simulink model "controller"  (R2023b)
settings: Solver=VariableStepAuto  StartTime=0.0  StopTime=10.0  RelTol=1e-3
undefined symbols (not defined in the file or in its folder): u0, u_lim_max, u_lim_min
settings Model: Creator=fabioschneider  LastModifiedBy=fabioschneider
settings DebuggingCC: ModelReferenceExtraNoncontSigs=none

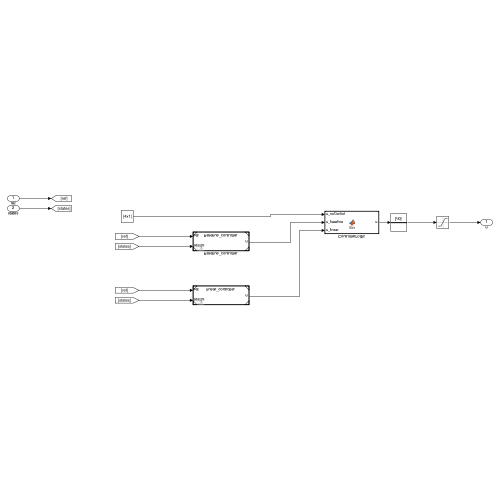
[thumbnail: Simulink's stored preview of the top-level diagram]
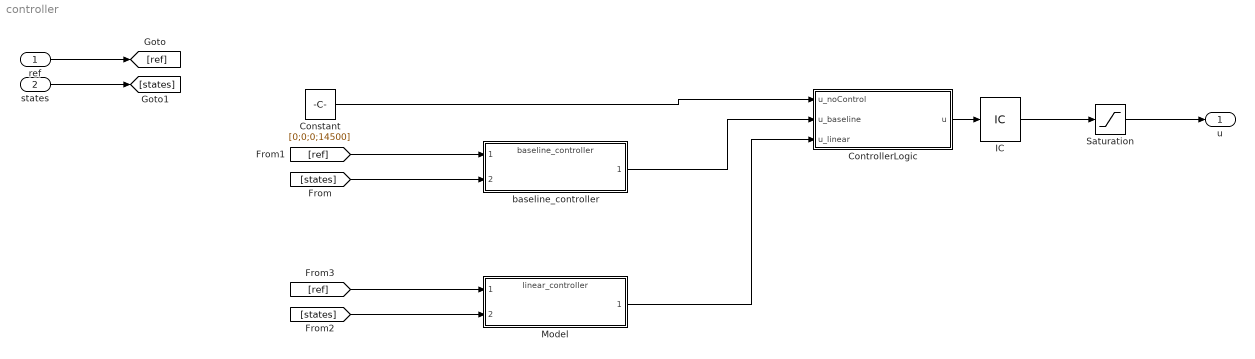
== system controller ==
  ref : Inport
  states : Inport  Port=2
  Constant : Constant  Value=[0;0;0;14500]  SampleTime=-1
  ControllerLogic : MATLAB Function  TreatAsAtomicUnit=on
  IC : InitialCondition  Value=u0
  Model : ModelReference  ModelNameDialog=linear_controller.slx  SimulationMode=Normal  ModelReferenceVersion=1.9
  Saturation : Saturate  UpperLimit=u_lim_max  LowerLimit=u_lim_min
  baseline_controller : ModelReference  ModelNameDialog=baseline_controller.slx  SimulationMode=Normal  ModelReferenceVersion=1.13
  u : Outport
  wires:
  ControllerLogic/1(u) -> IC/1
  Constant/1 -> ControllerLogic/1(u_noControl)
  baseline_controller/1 -> ControllerLogic/2(u_baseline)
  ref/1 -> [ref]
  states/1 -> [states]
  [states] -> baseline_controller/2
  [ref] -> baseline_controller/1
  Model/1 -> ControllerLogic/3(u_linear)
  IC/1 -> Saturation/1
  [ref] -> Model/1
  [states] -> Model/2
  Saturation/1 -> u/1

== matlab function controller/ControllerLogic ==
  data: u_noControl input; u output; u_baseline input; u_linear input; activeController parameter
function u = fcn(u_noControl, u_baseline, u_linear, activeController)

u = controller_logic(u_noControl, u_baseline, u_linear, activeController);
